simulink model "prj_v2_sb"  (R2022a)
settings: Solver=ode15s  StartTime=0.0  StopTime=20  FixedStep=0.1  RelTol=1e-3
model workspace (MAT data in the model file):
  interface_msg1 = Simulink.Bus
  interface_msg1.Alignment = -1
  interface_msg1.PreserveElementDimensions = 0
  interface_msg1.Elements_internal(1) = Simulink.BusElement
  interface_msg1.Elements_internal(1).Min_internal = -100
  interface_msg1.Elements_internal(1).Max_internal = 100
  interface_msg1.Elements_internal(1).DimensionsMode = 'Fixed'
  interface_msg1.Elements_internal(1).SamplingMode = 'Sample based'
  interface_msg1.Elements_internal(1).SampleTime = -1
  interface_msg1.Elements_internal(1).Name = 'x1'
  interface_msg1.Elements_internal(1).DataType_internal = 'int32'
  interface_msg1.Elements_internal(1).Complexity = 'real'
  interface_msg1.Elements_internal(1).Dimensions = 1
  interface_msg1.Elements_internal(2) = Simulink.BusElement
  interface_msg1.Elements_internal(2).Min_internal = -100
  interface_msg1.Elements_internal(2).Max_internal = 100
  interface_msg1.Elements_internal(2).DimensionsMode = 'Fixed'
  interface_msg1.Elements_internal(2).SamplingMode = 'Sample based'
  interface_msg1.Elements_internal(2).SampleTime = -1
  interface_msg1.Elements_internal(2).Name = 'y1'
  interface_msg1.Elements_internal(2).DataType_internal = 'int32'
  interface_msg1.Elements_internal(2).Complexity = 'real'
  interface_msg1.Elements_internal(2).Dimensions = 1
  interface_msg1.Elements_internal(3) = Simulink.BusElement
  interface_msg1.Elements_internal(3).Min_internal = -100
  interface_msg1.Elements_internal(3).Max_internal = 100
  interface_msg1.Elements_internal(3).DimensionsMode = 'Fixed'
  interface_msg1.Elements_internal(3).SamplingMode = 'Sample based'
  interface_msg1.Elements_internal(3).SampleTime = -1
  interface_msg1.Elements_internal(3).Name = 'dir1'
  interface_msg1.Elements_internal(3).DataType_internal = 'int32'
  interface_msg1.Elements_internal(3).Complexity = 'real'
  interface_msg1.Elements_internal(3).Dimensions = 1
  interface_msg1.DataScope = 'Auto'
  interface_msg2 = Simulink.Bus
  interface_msg2.Alignment = -1
  interface_msg2.PreserveElementDimensions = 0
  interface_msg2.Elements_internal(1) = Simulink.BusElement
  interface_msg2.Elements_internal(1).Min_internal = -100
  interface_msg2.Elements_internal(1).Max_internal = 100
  interface_msg2.Elements_internal(1).DimensionsMode = 'Fixed'
  interface_msg2.Elements_internal(1).SamplingMode = 'Sample based'
  interface_msg2.Elements_internal(1).SampleTime = -1
  interface_msg2.Elements_internal(1).Name = 'x2'
  interface_msg2.Elements_internal(1).DataType_internal = 'int32'
  interface_msg2.Elements_internal(1).Complexity = 'real'
  interface_msg2.Elements_internal(1).Dimensions = 1
  interface_msg2.Elements_internal(2) = Simulink.BusElement
  interface_msg2.Elements_internal(2).Min_internal = -100
  interface_msg2.Elements_internal(2).Max_internal = 100
  interface_msg2.Elements_internal(2).DimensionsMode = 'Fixed'
  interface_msg2.Elements_internal(2).SamplingMode = 'Sample based'
  interface_msg2.Elements_internal(2).SampleTime = -1
  interface_msg2.Elements_internal(2).Name = 'y2'
  interface_msg2.Elements_internal(2).DataType_internal = 'int32'
  interface_msg2.Elements_internal(2).Complexity = 'real'
  interface_msg2.Elements_internal(2).Dimensions = 1
  interface_msg2.Elements_internal(3) = Simulink.BusElement
  interface_msg2.Elements_internal(3).Min_internal = -100
  interface_msg2.Elements_internal(3).Max_internal = 100
  interface_msg2.Elements_internal(3).DimensionsMode = 'Fixed'
  interface_msg2.Elements_internal(3).SamplingMode = 'Sample based'
  interface_msg2.Elements_internal(3).SampleTime = -1
  interface_msg2.Elements_internal(3).Name = 'dir2'
  interface_msg2.Elements_internal(3).DataType_internal = 'int32'
  interface_msg2.Elements_internal(3).Complexity = 'real'
  interface_msg2.Elements_internal(3).Dimensions = 1
  interface_msg2.DataScope = 'Auto'
undefined symbols (not defined in the file): airplane2, msg, sigbuilder_block
settings Model: Creator=Iran  LastModifiedBy=FtmAh
settings SolverCC: AlgebraicLoopSolver=TrustRegion
settings DebuggingCC: UnconnectedInputMsg=warning  UnconnectedOutputMsg=warning  UnconnectedLineMsg=warning  SFMachineParentedDataDiag=warning
settings RTWCC: DLArmComputeVersion=19.05
settings ConfigComp: CovEnable=on  RecordCoverage=on  CovModelRefEnable=on  DVTestSuiteOptimization=Auto  DVDetectOutOfBounds=on  DVModelReferenceHarness=on  DVHarnessSource=Signal Editor

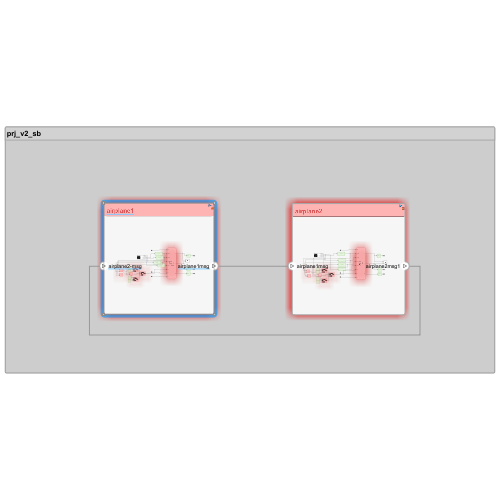
[thumbnail: Simulink's stored preview of the top-level diagram]
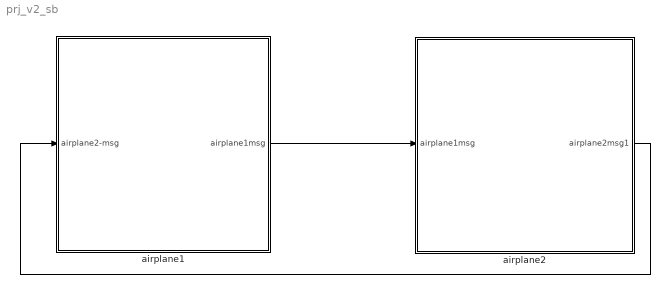
== system prj_v2_sb ==
  airplane1 : Subsystem
      settings: PortSchema="{\"entries\":[{\"content\":{\"headerSize\":26,\"margin\":15,\"minimumSpacing\":25,\"sides\":[{\"content\":{\"connectorIds\":[\"In1\"]},\"type\":\"ConnectorPlacement.EquallySpacedRectSide\",\"uuid\":\"381f2f55-2706-4a20-9b5c-d1d238ade6d6\"},{\"content\":{\"connectorIds\":[\"Out1\"],\"side\":\"RIGHT\"},\"type\":\"ConnectorPlacement.EquallySpacedRectSide\",\"uuid\":\"25d2ce27-d2f9-4747-86b3-2bcde07e6841\"},{\"content\":{\"connectorIds\":[],\"side\":\"TOP\"},\"type\":\"ConnectorPlacement.EquallySpacedRectSide\",\"uuid\":\"070681d8-a2bf-493e-aa62-f3e5dae2f343\"},{\"content\":{\"connectorIds\":[],\"side\":\"HIDDEN\"},\"type\":\"ConnectorPlacement.EquallySpacedRectSide\",\"uuid\":\"a3f7a84e-f675-4776-92e7-f80ce261eaa3\"}]},\"type\":\"ConnectorPlacement.EquallySpacedConnector\",\"uuid\":\"2503d3e3-c5a9-4ee9-9c8f-f126b5cdcb6a\"}],\"packageUris\":[\"http://schema.mathworks.com/mf0/Connector/R2020b\"],\"version\":\"1.0\"}"
  airplane2 : Subsystem
      settings: PortSchema="{\"entries\":[{\"content\":{\"headerSize\":26,\"margin\":15,\"minimumSpacing\":25,\"sides\":[{\"content\":{\"connectorIds\":[\"In1\"]},\"type\":\"ConnectorPlacement.EquallySpacedRectSide\",\"uuid\":\"381f2f55-2706-4a20-9b5c-d1d238ade6d6\"},{\"content\":{\"connectorIds\":[\"Out1\"],\"side\":\"RIGHT\"},\"type\":\"ConnectorPlacement.EquallySpacedRectSide\",\"uuid\":\"25d2ce27-d2f9-4747-86b3-2bcde07e6841\"},{\"content\":{\"connectorIds\":[],\"side\":\"TOP\"},\"type\":\"ConnectorPlacement.EquallySpacedRectSide\",\"uuid\":\"070681d8-a2bf-493e-aa62-f3e5dae2f343\"},{\"content\":{\"connectorIds\":[],\"side\":\"HIDDEN\"},\"type\":\"ConnectorPlacement.EquallySpacedRectSide\",\"uuid\":\"a3f7a84e-f675-4776-92e7-f80ce261eaa3\"}]},\"type\":\"ConnectorPlacement.EquallySpacedConnector\",\"uuid\":\"2503d3e3-c5a9-4ee9-9c8f-f126b5cdcb6a\"}],\"packageUris\":[\"http://schema.mathworks.com/mf0/Connector/R2020b\"],\"version\":\"1.0\"}"
  wires:
  airplane1/1(airplane1msg) -> airplane2/1(airplane1msg)
  airplane2/1(airplane2msg1) -> airplane1/1(airplane2-msg)

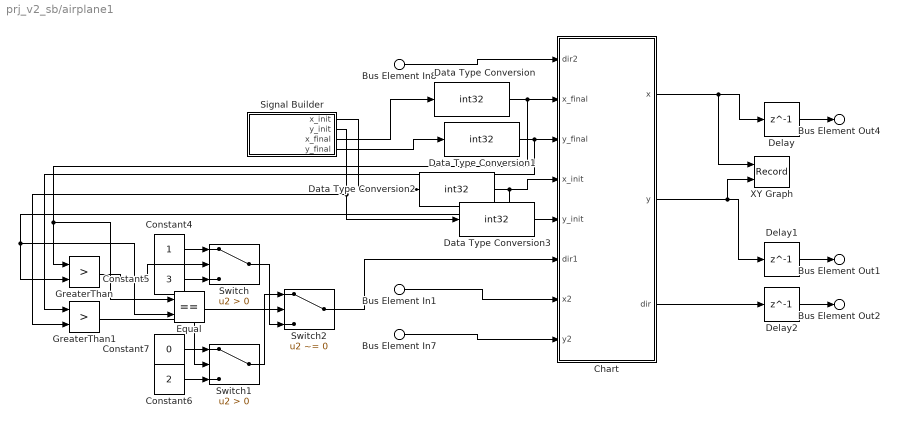
== system prj_v2_sb/airplane1 ==
  Bus Element In1 : Inport  PortName=airplane2-msg  Element=x2
  Bus Element In7 : Inport  PortName=airplane2-msg  Element=y2
  Bus Element In8 : Inport  PortName=airplane2-msg  Element=dir2
  Chart : Stateflow chart  TreatAsAtomicUnit=on
  Constant4 : Constant  OutDataTypeStr=uint32
  Constant5 : Constant  Value=3  OutDataTypeStr=uint32
  Constant6 : Constant  Value=2  OutDataTypeStr=uint32
  Constant7 : Constant  Value=0  OutDataTypeStr=uint32
  Data Type Conversion{,1..3} (4 alike) : DataTypeConversion  OutDataTypeStr=int32  SaturateOnIntegerOverflow=off  RndMeth=Floor
  Delay : Delay  DelayLength=1
  Delay1 : Delay  DelayLength=1
  Delay2 : Delay  DelayLength=1
  Equal : RelationalOperator  Operator===  OutDataTypeStr=boolean  RndMeth=Simplest  InputSameDT=off
  GreaterThan : RelationalOperator  Operator=>  OutDataTypeStr=boolean  RndMeth=Simplest  InputSameDT=off
  GreaterThan1 : RelationalOperator  Operator=>  OutDataTypeStr=boolean  RndMeth=Simplest  InputSameDT=off
  Signal Builder : Subsystem  Tag=STV Subsys  LoadFcn=sigbuilder_block('load');  StartFcn=sigbuilder_block('start');  StopFcn=sigbuilder_block('stop');  ClipboardFcn=sigbuilder_block('clipboard');  mask(Sigbuilder block){tuvar=[0:10]}
      mask help: Simulink:masks:SigbuilderBlock_MD
      mask init:
      | if ~strcmp(get_param(bdroot(gcbh),'SimulationStatus'),'stopped') tuvar = sigbuilder_block('maskInit'); end
      settings: CopyFcn=sigbuilder_block('copy');  DeleteFcn=sigbuilder_block('delete');  ModelCloseFcn=sigbuilder_block('modelClose');  PreSaveFcn=sigbuilder_block('preSave');  PauseFcn=sigbuilder_block('pause');  ContinueFcn=sigbuilder_block('continue');  NameChangeFcn=sigbuilder_block('namechange');  OpenFcn=sigbuilder_block('open',[351.75 138 550.5 355.5 ]);  CloseFcn=sigbuilder_block('close');
      mask Display: plot(0, 0, 100, 100,[2, 2, 32, 32, 2], [68, 8, 8, 68, 68],[32, 2], [38, 38], [32, 19, 2],[53, 60, 44], [32, 17, 17, 2],[16, 16, 31, 31]);txt = getActiveGroup(gcbh);text(2, 100, txt,'verticalAlignment', 'top');
  Switch : Switch  Criteria=u2 > Threshold  SaturateOnIntegerOverflow=off  InputSameDT=off
  Switch1 : Switch  Criteria=u2 > Threshold  SaturateOnIntegerOverflow=off  InputSameDT=off
  Switch2 : Switch  Criteria=u2 ~= 0  OutDataTypeStr=int32  SaturateOnIntegerOverflow=off  InputSameDT=off
  XY Graph : Record  FileSettingsInternal="{\"entries\":[{\"content\":{\"excelSettings\":{\"content\":{},\"type\":\"Streamout.ExcelSettings\"}},\"type\":\"Streamout.FileSettingStorage\",\"uuid\":\"259eee5e-7291-4375-968a-4c28429b4305\"}],\"packageUris\":[\"http://schema.mathworks.com/mf0/streamout_blocks/R2020a\"],\"version\":\"1.0\"}"  Layout=[1 1]  SignalsInternal="{\"entries\":[{\"content\":{\"signals\":[{\"content\":{\"blockPath\":[\"prj_v2_sb/airplane1/XY Graph\"],\"channel\":[],\"dimensions\":[1],\"domain\":\"prj_v2_sb/airplane1/XY Graph\",\"lineColor\":\"#a2142f\",\"plots\":[1],\"port\":1,\"sid\":[\"\"],\"signalID\":8888,\"signalName\":\"Chart:1\"},\"type\":\"RecordBlkView.Signal\",\"uuid\":\"75ce961a-c881-462b-a8e4-1a08f6d6652d\"},{\"content\":{\"blockPath\":[\"prj_v2_sb/airplane1/XY Graph\"],\"channel\":[],\"dimensions\":[1],\"domain\":\"prj_v2_sb/airplane1/XY Graph\",\"lineColor\":\"#139fff\",\"plots\":[1],\"port\":2,\"sid\":[\"\"],\"signalID\":8892,\"signalName\":\"Chart:2\"},\"type\":\"RecordBlkView.Signal\",\"uuid\":\"2dc82c44-cf4f-4d0c-a74d-5109abd042be\"}]},\"type\":\"RecordBlkView.InputSignals\",\"uuid\":\"799a1abc-ed27-4f4a-9f71-43168998b88a\"}],\"packageUris\":[\"http://schema.mathworks.com/mf0/streamout_blocks/R2020a\"],\"version\":\"1.0\"}"  VisualizationBindings="{\"xyplotplugin\":{\"info\":[{\"series\":[{\"bindingParametersList\":[{\"parameter\":\"X-Axis\",\"signalID\":8888,\"signalName\":\"Chart:1\"},{\"parameter\":\"Y-Axis\",\"signalID\":8892,\"signalName\":\"Chart:2\"}],\"seriesID\":35656}],\"subplotID\":1}]}}"  CompatibilityTag=XY
  Bus Element Out4 : Outport  PortName=airplane1msg  Element=x1
  Bus Element Out1 : Outport  PortName=airplane1msg  Element=y1
  Bus Element Out2 : Outport  PortName=airplane1msg  Element=dir1
  wires:
  Chart/3(dir) -> Delay2/1
  Bus Element In7/1 -> Chart/8(y2)
  Chart/2(y) -> XY Graph/2, Delay1/1
  Signal Builder/3(x_final) -> Data Type Conversion/1
  Bus Element In8/1 -> Chart/1(dir2)
  Chart/1(x) -> XY Graph/1, Delay/1
  Bus Element In1/1 -> Chart/7(x2)
  Delay/1 -> Bus Element Out4/1
  Delay1/1 -> Bus Element Out1/1
  Delay2/1 -> Bus Element Out2/1
  Constant5/1 -> Switch/3
  GreaterThan/1 -> Switch/2
  Constant4/1 -> Switch/1
  Constant7/1 -> Switch1/1
  Constant6/1 -> Switch1/3
  Switch2/1 -> Chart/6(dir1)
  GreaterThan1/1 -> Switch1/2
  Equal/1 -> Switch2/2
  Switch1/1 -> Switch2/1
  Switch/1 -> Switch2/3
  Data Type Conversion/1 -> Equal/1, GreaterThan/1, Chart/2(x_final)
  Data Type Conversion1/1 -> GreaterThan1/1, Chart/3(y_final)
  Signal Builder/4(y_final) -> Data Type Conversion1/1
  Data Type Conversion2/1 -> Equal/2, GreaterThan/2, Chart/4(x_init)
  Signal Builder/1(x_init) -> Data Type Conversion2/1
  Data Type Conversion3/1 -> Chart/5(y_init)
  Signal Builder/2(y_init) -> GreaterThan1/2, Data Type Conversion3/1

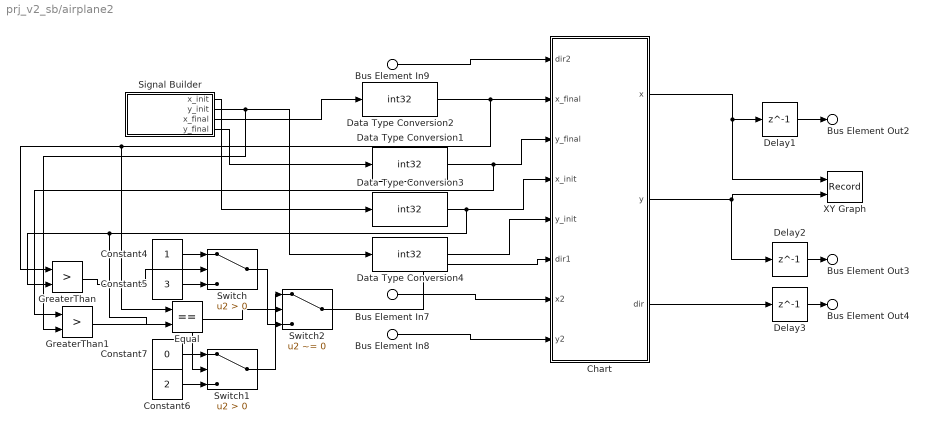
== system prj_v2_sb/airplane2 ==
  Bus Element In7 : Inport  PortName=airplane1msg  Element=x1
  Bus Element In8 : Inport  PortName=airplane1msg  Element=y1
  Bus Element In9 : Inport  PortName=airplane1msg  Element=dir1
  Chart : Stateflow chart  TreatAsAtomicUnit=on
  Constant4 : Constant  OutDataTypeStr=uint32
  Constant5 : Constant  Value=3  OutDataTypeStr=uint32
  Constant6 : Constant  Value=2  OutDataTypeStr=uint32
  Constant7 : Constant  Value=0  OutDataTypeStr=uint32
  Data Type Conversion{1..4} (4 alike) : DataTypeConversion  OutDataTypeStr=int32  SaturateOnIntegerOverflow=off  RndMeth=Floor
  Delay1 : Delay  DelayLength=1
  Delay2 : Delay  DelayLength=1
  Delay3 : Delay  DelayLength=1
  Equal : RelationalOperator  Operator===  OutDataTypeStr=boolean  RndMeth=Simplest  InputSameDT=off
  GreaterThan : RelationalOperator  Operator=>  OutDataTypeStr=boolean  RndMeth=Simplest  InputSameDT=off
  GreaterThan1 : RelationalOperator  Operator=>  OutDataTypeStr=boolean  RndMeth=Simplest  InputSameDT=off
  Signal Builder : Subsystem  Tag=STV Subsys  LoadFcn=sigbuilder_block('load');  StartFcn=sigbuilder_block('start');  StopFcn=sigbuilder_block('stop');  ClipboardFcn=sigbuilder_block('clipboard');  mask(Sigbuilder block){tuvar=[0:10]}
      mask help: Simulink:masks:SigbuilderBlock_MD
      mask init:
      | if ~strcmp(get_param(bdroot(gcbh),'SimulationStatus'),'stopped') tuvar = sigbuilder_block('maskInit'); end
      settings: CopyFcn=sigbuilder_block('copy');  DeleteFcn=sigbuilder_block('delete');  ModelCloseFcn=sigbuilder_block('modelClose');  PreSaveFcn=sigbuilder_block('preSave');  PauseFcn=sigbuilder_block('pause');  ContinueFcn=sigbuilder_block('continue');  NameChangeFcn=sigbuilder_block('namechange');  OpenFcn=sigbuilder_block('open',[351.75 138 550.5 355.5 ]);  CloseFcn=sigbuilder_block('close');
      mask Display: plot(0, 0, 100, 100,[2, 2, 32, 32, 2], [68, 8, 8, 68, 68],[32, 2], [38, 38], [32, 19, 2],[53, 60, 44], [32, 17, 17, 2],[16, 16, 31, 31]);txt = getActiveGroup(gcbh);text(2, 100, txt,'verticalAlignment', 'top');
  Switch : Switch  Criteria=u2 > Threshold  SaturateOnIntegerOverflow=off  InputSameDT=off
  Switch1 : Switch  Criteria=u2 > Threshold  SaturateOnIntegerOverflow=off  InputSameDT=off
  Switch2 : Switch  Criteria=u2 ~= 0  OutDataTypeStr=int32  SaturateOnIntegerOverflow=off  InputSameDT=off
  XY Graph : Record  FileSettingsInternal="{\"entries\":[{\"content\":{\"excelSettings\":{\"content\":{},\"type\":\"Streamout.ExcelSettings\"}},\"type\":\"Streamout.FileSettingStorage\",\"uuid\":\"aa3f6859-6199-4ebf-9d41-a61cce50d281\"}],\"packageUris\":[\"http://schema.mathworks.com/mf0/streamout_blocks/R2020a\"],\"version\":\"1.0\"}"  Layout=[1 1]  SignalsInternal="{\"entries\":[{\"content\":{\"signals\":[{\"content\":{\"blockPath\":[\"prj_v2_sb/airplane2/XY Graph\"],\"channel\":[],\"dimensions\":[1],\"domain\":\"prj_v2_sb/airplane2/XY Graph\",\"lineColor\":\"#a2142f\",\"plots\":[1],\"port\":1,\"sid\":[\"\"],\"signalID\":8896,\"signalName\":\"Chart:1\"},\"type\":\"RecordBlkView.Signal\",\"uuid\":\"11e98f95-e29f-45c0-9cfd-6f0bf2296910\"},{\"content\":{\"blockPath\":[\"prj_v2_sb/airplane2/XY Graph\"],\"channel\":[],\"dimensions\":[1],\"domain\":\"prj_v2_sb/airplane2/XY Graph\",\"lineColor\":\"#139fff\",\"plots\":[1],\"port\":2,\"sid\":[\"\"],\"signalID\":8900,\"signalName\":\"Chart:2\"},\"type\":\"RecordBlkView.Signal\",\"uuid\":\"2686b6d3-6614-4aad-b2b0-19b9d21b7d6a\"}]},\"type\":\"RecordBlkView.InputSignals\",\"uuid\":\"5b103666-3157-4f53-8e40-96c3a53350e2\"}],\"packageUris\":[\"http://schema.mathworks.com/mf0/streamout_blocks/R2020a\"],\"version\":\"1.0\"}"  VisualizationBindings="{\"xyplotplugin\":{\"info\":[{\"series\":[{\"bindingParametersList\":[{\"parameter\":\"X-Axis\",\"signalID\":8896,\"signalName\":\"Chart:1\"},{\"parameter\":\"Y-Axis\",\"signalID\":8900,\"signalName\":\"Chart:2\"}],\"seriesID\":52745}],\"subplotID\":1}]}}"  CompatibilityTag=XY
  Bus Element Out2 : Outport  PortName=airplane2msg1  Element=x2
  Bus Element Out3 : Outport  PortName=airplane2msg1  Element=y2
  Bus Element Out4 : Outport  PortName=airplane2msg1  Element=dir2
  wires:
  Chart/3(dir) -> Delay3/1
  Bus Element In8/1 -> Chart/8(y2)
  Chart/2(y) -> XY Graph/2, Delay2/1
  Bus Element In9/1 -> Chart/1(dir2)
  Chart/1(x) -> XY Graph/1, Delay1/1
  Bus Element In7/1 -> Chart/7(x2)
  Delay1/1 -> Bus Element Out2/1
  Delay2/1 -> Bus Element Out3/1
  Delay3/1 -> Bus Element Out4/1
  Switch2/1 -> Chart/6(dir1)
  GreaterThan1/1 -> Switch1/2
  Constant6/1 -> Switch1/3
  Constant7/1 -> Switch1/1
  Constant4/1 -> Switch/1
  Constant5/1 -> Switch/3
  GreaterThan/1 -> Switch/2
  Equal/1 -> Switch2/2
  Switch/1 -> Switch2/3
  Switch1/1 -> Switch2/1
  Signal Builder/3(x_final) -> Data Type Conversion2/1
  Data Type Conversion2/1 -> GreaterThan/1, Equal/1, Chart/2(x_final)
  Data Type Conversion1/1 -> GreaterThan1/1, Chart/3(y_final)
  Signal Builder/4(y_final) -> Data Type Conversion1/1
  Data Type Conversion3/1 -> GreaterThan/2, Equal/2, Chart/4(x_init)
  Signal Builder/1(x_init) -> Data Type Conversion3/1
  Data Type Conversion4/1 -> Chart/5(y_init)
  Signal Builder/2(y_init) -> GreaterThan1/2, Data Type Conversion4/1

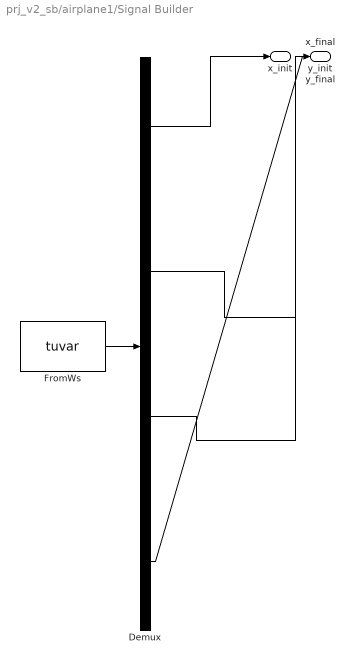
== system prj_v2_sb/airplane1/Signal Builder ==
  Demux : Demux  Tag=STV Demux
      settings: DisplayOption=none
  FromWs : FromWorkspace  Tag=STV FromWs  VariableName=tuvar
      SigBuilderData=|
      | common.afterFinalStr = 'Extrapolate'
      | common.sampleTime = 0
      | dataSet.timeRange = [0 20]
      | dataSet.name = 'Sheet1'
      | sbobj.Groups.Name = 'Sheet1'
      | sbobj.Groups.Signals(1).Name = 'x_init'
      | sbobj.Groups.Signals(1).XData = [0 20]
      | sbobj.Groups.Signals(1).YData = [2 2]
      | sbobj.Groups.Signals(2).Name = 'y_init'
      | sbobj.Groups.Signals(2).XData = [0 20]
      | sbobj.Groups.Signals(2).YData = [3 3]
      | sbobj.Groups.Signals(3).Name = 'x_final'
      | sbobj.Groups.Signals(3).XData = [0 20]
      | sbobj.Groups.Signals(3).YData = [5 5]
      | sbobj.Groups.Signals(4).Name = 'y_final'
      | sbobj.Groups.Signals(4).XData = [0 20]
      | sbobj.Groups.Signals(4).YData = [3 3]
      | sbobj.Groups.TimeRange = [0 20]
  x_init : Outport  Tag=STV Outport
  y_init : Outport  Tag=STV Outport  Port=2
  x_final : Outport  Tag=STV Outport  Port=3
  y_final : Outport  Tag=STV Outport  Port=4
  wires:
  Demux/1 -> x_init/1
  FromWs/1 -> Demux/1
  Demux/2 -> y_init/1
  Demux/3 -> x_final/1
  Demux/4 -> y_final/1

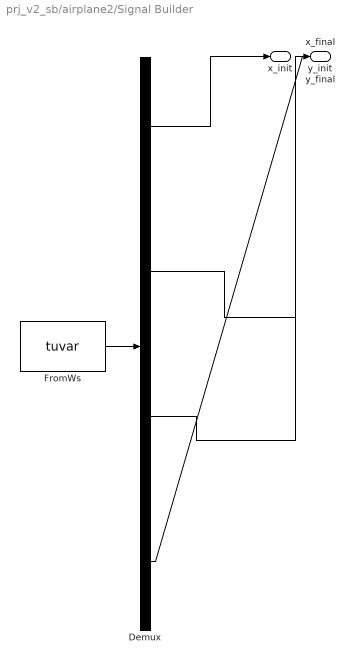
== system prj_v2_sb/airplane2/Signal Builder ==
  Demux : Demux  Tag=STV Demux
      settings: DisplayOption=none
  FromWs : FromWorkspace  Tag=STV FromWs  VariableName=tuvar
      SigBuilderData=|
      | common.afterFinalStr = 'Extrapolate'
      | common.sampleTime = 0
      | dataSet.timeRange = [0 20]
      | dataSet.name = 'Sheet1'
      | sbobj.Groups.Name = 'Sheet1'
      | sbobj.Groups.Signals(1).Name = 'x_init'
      | sbobj.Groups.Signals(1).XData = [0 20]
      | sbobj.Groups.Signals(1).YData = [4 4]
      | sbobj.Groups.Signals(2).Name = 'y_init'
      | sbobj.Groups.Signals(2).XData = [0 20]
      | sbobj.Groups.Signals(2).YData = [3 3]
      | sbobj.Groups.Signals(3).Name = 'x_final'
      | sbobj.Groups.Signals(3).XData = [0 20]
      | sbobj.Groups.Signals(3).YData = [1 1]
      | sbobj.Groups.Signals(4).Name = 'y_final'
      | sbobj.Groups.Signals(4).XData = [0 20]
      | sbobj.Groups.Signals(4).YData = [3 3]
      | sbobj.Groups.TimeRange = [0 40]
  x_init : Outport  Tag=STV Outport
  y_init : Outport  Tag=STV Outport  Port=2
  x_final : Outport  Tag=STV Outport  Port=3
  y_final : Outport  Tag=STV Outport  Port=4
  wires:
  Demux/1 -> x_init/1
  FromWs/1 -> Demux/1
  Demux/2 -> y_init/1
  Demux/3 -> x_final/1
  Demux/4 -> y_final/1

== stateflow chart prj_v2_sb/airplane1/Chart ==
  settings: updateMethod=CONTINUOUS
  state initial
    during:
    s_dot = 1;
  state horizontal_move
    during:
    s_dot = 1;
  state vertical_move
    during:
    s_dot = 1;
  (default) -> initial : {s = 0 ; x = x_init; y = y_init; dir = dir1;}
  horizontal_move -> horizontal_move [order 3] : [y_final == y && x_final ~= x && s >= 1]{s = 0; y = y + 1; dir = 0}
  initial -> horizontal_move [order 3] : [x_final ~= x && s >= 0 && ~(x2 == x + 1 && y2 == y + 1 && dir2 == 2 && x_final > x) && ~(x == x2 + 1 && y2 == y + 1 && dir2 == 2 && x_final < x) && ~(x2 == x + 1 && y == y2 + 1 && dir2 == 0 && x_final > x) && ~(x == x2 + 1 && y == y2 + 1 && dir2 == 0 && x_final < x) && ~(y2 == y && x2 == x + 2 && dir2 == 3 && x_final > x) && ~(y2 == y && x2 == x + 1 && dir2 == 3 && x_final > x)]{s = 0;}
  initial -> initial [order 2] : [y_final == y && x_final == x && s >= 1]{dir = 4; s = 0}
  horizontal_move -> horizontal_move [order 1] : [x_final < x && s >= 1 && ~(x == x2 + 1 && y == y2 + 1 && dir2 == 0 && x_final < x) && ~(x == x2 + 1 && y2 == y + 1 && dir2 == 2 && x_final < x) ]{s = 0 ; x = x - 1; dir = 3}
  horizontal_move -> initial [order 4] : [s >= 1]{s = 0}
  horizontal_move -> horizontal_move [order 2] : [x_final > x && s>=1 &&  ~(x2 == x + 1 && y2 == y + 1 && dir2 == 2) && ~(x2 == x + 1 && y == y2 + 1 && dir2 == 0) && ~(y2 == y && x2 == x + 2 && dir2 == 3) && ~(y2 == y && x2 == x + 1 && dir2 == 3)]{s = 0;x = x + 1; dir = 1}
  initial -> vertical_move [order 1] : [y_final ~= y && s >= 0 && ~(x2 == x && y2 == y + 2 && dir2 == 2 && y_final > y) && ~(x2 == x && y2 == y + 1 && dir2 == 2 && y_final > y)]{s=0}
  vertical_move -> initial [order 4] : [s >= 1]{s = 0}
  vertical_move -> vertical_move [order 1] : [y_final < y && s >=1]{s=0;y=y-1; dir = 2}
  vertical_move -> vertical_move [order 2] : [y_final > y && s >=1 && ~(x2 == x && y2 == y + 2 && dir2 == 2)  && ~(x2 == x && y2 == y + 1 && dir2 == 2)]{s = 0; y = y + 1; dir = 0}
  vertical_move -> vertical_move [order 3] : [ x_final == x && y_final ~= y && s >=1]{s = 0; x = x + 1; dir = 1}
  data: dir2 input int32; x_final input int32; y_final input int32; x_init input int32; x output int32; y output int32; y_init input int32; dir1 input int32; x2 input int32; y2 input int32; s local; dir output int32
  data s settings: updateMethod=SF_CONTINUOUS_TIME_DATA

== stateflow chart prj_v2_sb/airplane2/Chart ==
  settings: updateMethod=CONTINUOUS
  state initial
    during:
    s_dot = 1;
  state horizontal_move
    during:
    s_dot = 1;
  state vertical_move
    during:
    s_dot = 1;
  (default) -> initial : {s = 0 ; x = x_init; y = y_init; dir = dir1;}
  horizontal_move -> horizontal_move [order 3] : [y_final == y && x_final ~= x &&  s >=1]{y = y + 1; dir = 0}
  initial -> initial [order 3] : [y_final == y && x_final == x && s >= 1]{dir = 4; s = 0}
  horizontal_move -> horizontal_move [order 1] : [x_final < x && s >=1 && ~(x == x2 + 1 && y == y2 + 1 && dir2 == 0) && ~(x == x2 + 1 && y2 == y + 1 && dir2 == 2) ]{s = 0 ; x = x - 1; dir = 3}
  initial -> horizontal_move [order 1] : [x_final ~= x && s >= 0 && ~(x2 == x + 1 && y2 == y + 1 && dir2 == 2 && x_final > x) && ~(x == x2 + 1 && y2 == y + 1 && dir2 == 2 && x_final < x) && ~(x2 == x + 1 && y == y2 + 1 && dir2 == 0 && x_final > x) && ~(x == x2 + 1 && y == y2 + 1 && dir2 == 0 && x_final < x) && ~(y2 == y && x2 == x + 2 && dir2 == 3 && x_final > x) && ~(y2 == y && x2 == x + 1 && dir2 == 3 && x_final > x)]{s = 0;}
  horizontal_move -> initial [order 4] : [s >= 1]{s = 0}
  horizontal_move -> horizontal_move [order 2] : [x_final > x && s>=1 && ~(x2 == x + 1 && y2 == y + 1 && dir2 == 2 && x_final > x) && ~(x2 == x + 1 && y == y2 + 1 && dir2 == 0 && x_final > x) && ~(y2 == y && x2 == x + 2 && dir2 == 3 && x_final > x) && ~(y2 == y && x2 == x + 1 && dir2 == 3 && x_final > x)]{s = 0; x = x + 1; dir = 1}
  initial -> vertical_move [order 2] : [y_final ~= y && s >= 0 && ~(x2 == x && y2 == y + 2 && dir2 == 2 && y_final > y) && ~(x2 == x && y2 == y + 1 && dir2 == 2 && y_final > y)]{s = 0}
  vertical_move -> initial [order 4] : [s >= 1]{s = 0}
  vertical_move -> vertical_move [order 1] : [y_final < y && s >=1]{s = 0; y = y - 1; dir = 2}
  vertical_move -> vertical_move [order 2] : [y_final > y && s >=1 && ~(x2 == x && y2 == y + 2 && dir2 == 2) && ~(x2 == x && y2 == y + 1 && dir2 == 2)]{s = 0; y = y + 1; dir = 0}
  vertical_move -> vertical_move [order 3] : [x_final == x && y_final ~= y &&  s >=1]{x = x + 1; dir = 1}
  data: dir2 input int32; x_final input int32; y_final input int32; x_init input int32; x output int32; y output int32; y_init input int32; dir1 input int32; x2 input int32; y2 input int32; s local; dir output int32
  data s settings: updateMethod=SF_CONTINUOUS_TIME_DATA
